simulink model "Part2_ASK"  (R2017a)
settings: Solver=VariableStepAuto  StartTime=0.0  StopTime=1  RelTol=1e-3
undefined symbols (not defined in the file): randseed
libraries: commrandsrc3 x1, commfilt2 x1
settings Model: Creator=Marine  LastModifiedBy=mhuynh7
settings SFSimCC: SimUseLocalCustomCode=on
settings RTWCC: RTWUseLocalCustomCode=on

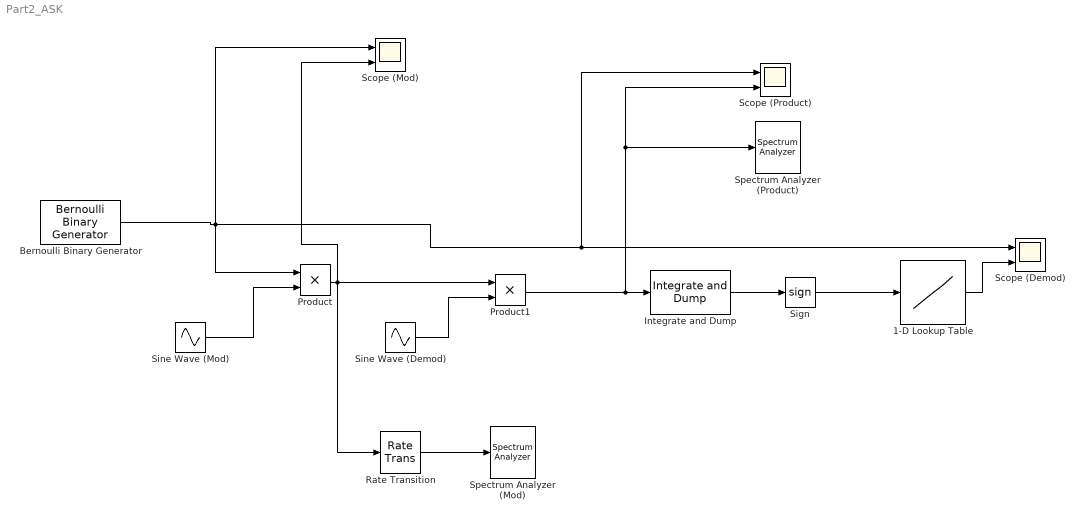
== system Part2_ASK ==
  1-D Lookup Table : Lookup_n-D  NumberOfTableDimensions=1  BreakpointsForDimension1=[-1,0,1]  Table=[0,0,1]  InternalRulePriority=Speed  RndMeth=Simplest  InputSameDT=on
  Bernoulli Binary Generator : commrandsrc3/Bernoulli Binary Generator  ProbabilityOfZero=0.5  SeedSource=Parameter  Seed=randseed  SampleTime=0.001  SamplesPerFrame=1  OutputDataType=double  SimulateUsing=Interpreted execution
  Integrate and Dump : commfilt2/Integrate and Dump  obssamples=8  offsetsamples=0  nodump=off  roundingMode=Floor  overflowMode=off  outputDataTypeStr=Inherit: Same as accumulator  outputLastDataTypeStr=Inherit: Same as accumulator
      settings: SourceProductName=Communications System Toolbox
  Product : Product
  Product1 : Product
  Rate Transition : RateTransition  OutPortSampleTime=0.5e-4
  Scope (Demod) : Scope  NumInputPorts=2
  Scope (Mod) : Scope  NumInputPorts=2
  Scope (Product) : Scope  NumInputPorts=2
  Sign : Signum
  Sine Wave (Demod) : Sin  SineType=Sample based  Samples=5000  SampleTime=1e-7
  Sine Wave (Mod) : Sin  SineType=Sample based  Samples=5000  SampleTime=1e-7
  Spectrum Analyzer (Mod) : SpectrumAnalyzer
  Spectrum Analyzer (Product) : SpectrumAnalyzer
  wires:
  Sine Wave (Mod)/1 -> Product/2
  Product/1 -> Scope (Mod)/2, Product1/1, Rate Transition/1
  Sine Wave (Demod)/1 -> Product1/2
  Rate Transition/1 -> Spectrum Analyzer (Mod)/1
  1-D Lookup Table/1 -> Scope (Demod)/2
  Sign/1 -> 1-D Lookup Table/1
  Bernoulli Binary Generator/1 -> Product/1, Scope (Mod)/1, Scope (Demod)/1, Scope (Product)/1
  Product1/1 -> Integrate and Dump/1, Spectrum Analyzer (Product)/1, Scope (Product)/2
  Integrate and Dump/1 -> Sign/1
